simulink model "TestWindRacingSimpleDynamicModelRealForce"  (R2022b)
settings: Solver=FixedStepAuto  StartTime=0.0  StopTime=137  FixedStep=simulator.TimeStep  RelTol=1e-3
undefined symbols (not defined in the file): simulator
settings Model: Creator=At  LastModifiedBy=ateay
settings SolverCC: ConcurrentTasks=on  AlgebraicLoopSolver=TrustRegion  InsertRTBMode=Never (minimum delay)
settings DataIOCC: ReturnWorkspaceOutputs=off
settings DebuggingCC: UnconnectedInputMsg=warning  UnconnectedOutputMsg=warning  UnconnectedLineMsg=warning  SFMachineParentedDataDiag=warning  ArithmeticOperatorsInVariantConditions=warning
settings ModelReferenceCC: EnableRefExpFcnMdlSchedulingChecks=on
settings SFSimCC: SimUseLocalCustomCode=off  CustomCodeUndefinedFunction=UseInterfaceOnly
settings RTWCC: RTWUseLocalCustomCode=off
settings CodeAppCC: StateflowObjectComments=on

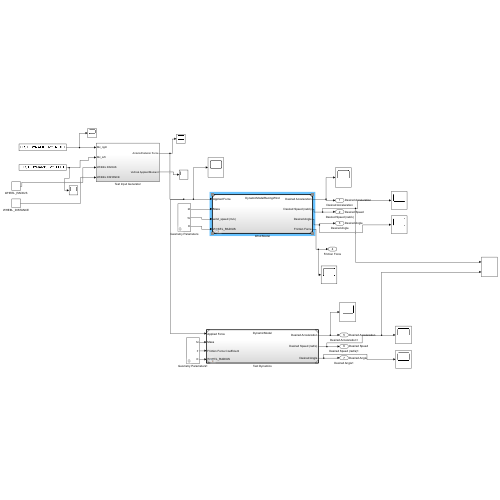
[thumbnail: Simulink's stored preview of the top-level diagram]
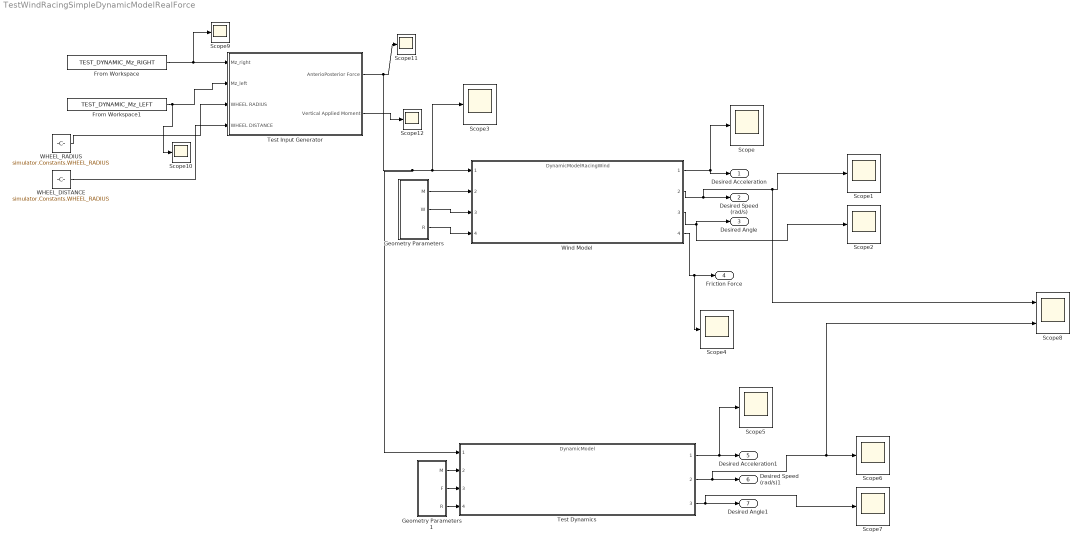
== system TestWindRacingSimpleDynamicModelRealForce ==
  From Workspace : FromWorkspace  VariableName=TEST_DYNAMIC_Mz_RIGHT
  From Workspace1 : FromWorkspace  VariableName=TEST_DYNAMIC_Mz_LEFT
  Geometry Parameters : Subsystem  mask{M=simulator.Sim.Dynamics.Mass, W=simulator.Sim.Dynamics.wind_speed, rR=simulator.Constants.WHEEL_RADIUS}
      mask prompts: M "Mass"; W "Wind"; rR "Radius"
      mask TypeOptions M: Mass/Value
      mask TypeOptions rR: rR/Value
  Geometry Parameters1 : Subsystem  mask{M=98, F=0.0138, rR=0.350}
      mask prompts: M "Mass"; F "Friction"; rR "Radius"
      mask TypeOptions M: Mass/Value
      mask TypeOptions F: Friction/Value
      mask TypeOptions rR: rR/Value
  Scope{,1..7,9..12} (12 alike) : Scope
  Scope8 : Scope  NumInputPorts=2
  "Test Dynamics " : ModelReference  ModelNameDialog=DynamicModel.slx  SimulationMode=Normal  ModelReferenceVersion=1.2
  Test Input Generator : Subsystem
  WHEEL_DISTANCE : Constant  Value=simulator.Constants.WHEEL_RADIUS
  WHEEL_RADIUS : Constant  Value=simulator.Constants.WHEEL_RADIUS
  Wind Model : ModelReference  ModelNameDialog=DynamicModelRacingWind.slx  SimulationMode=Normal  ModelReferenceVersion=1.17
  Desired Acceleration : Outport  SignalName=Desired Acceleration
  Desired Speed (rad/s) : Outport  Port=2  SignalName=Desired Speed
  Desired Angle : Outport  Port=3  SignalName=Desired Angle
  Friction Force : Outport  Port=4
  Desired Acceleration1 : Outport  Port=5  SignalName=Desired Acceleration
  Desired Speed (rad/s)1 : Outport  Port=6  SignalName=Desired Speed
  Desired Angle1 : Outport  Port=7  SignalName=Desired Angle
  wires:
  Wind Model/3 -> Desired Angle/1, Scope2/1
  Wind Model/2 -> Scope8/1, Scope1/1, Desired Speed (rad/s)/1
  Wind Model/1 -> Desired Acceleration/1, Scope/1
  Geometry Parameters/1(M) -> Wind Model/2
  Geometry Parameters/2(W) -> Wind Model/3
  Geometry Parameters/3(R) -> Wind Model/4
  Wind Model/4 -> Scope4/1, Friction Force/1
  Test Input Generator/1(AnterioPosterior Force) -> "Test Dynamics "/1, Wind Model/1, Scope3/1, Scope11/1
  "Test Dynamics "/3 -> Scope7/1, Desired Angle1/1
  "Test Dynamics "/2 -> Scope8/2, Scope6/1, Desired Speed (rad/s)1/1
  "Test Dynamics "/1 -> Scope5/1, Desired Acceleration1/1
  Geometry Parameters1/1(M) -> "Test Dynamics "/2
  Geometry Parameters1/2(F) -> "Test Dynamics "/3
  Geometry Parameters1/3(R) -> "Test Dynamics "/4
  WHEEL_RADIUS/1 -> Test Input Generator/3(WHEEL RADIUS)
  WHEEL_DISTANCE/1 -> Test Input Generator/4(WHEEL DISTANCE)
  Test Input Generator/2(Vertical Applied Moment) -> Scope12/1
  From Workspace/1 -> Scope9/1, Test Input Generator/1(Mz_right)
  From Workspace1/1 -> Scope10/1, Test Input Generator/2(Mz_left)

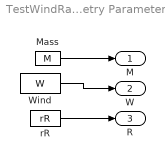
== system TestWindRacingSimpleDynamicModelRealForce/Geometry Parameters ==
  Mass : Constant  Value=M
  Wind : Constant  Value=W
  rR : Constant  Value=rR
  M : Outport
  W : Outport  Port=2
  R : Outport  Port=3
  wires:
  Wind/1 -> W/1
  Mass/1 -> M/1
  rR/1 -> R/1

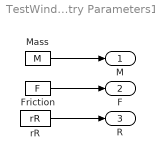
== system TestWindRacingSimpleDynamicModelRealForce/Geometry Parameters1 ==
  Friction : Constant  Value=F
  Mass : Constant  Value=M
  rR : Constant  Value=rR
  M : Outport
  F : Outport  Port=2
  R : Outport  Port=3
  wires:
  Friction/1 -> F/1
  Mass/1 -> M/1
  rR/1 -> R/1

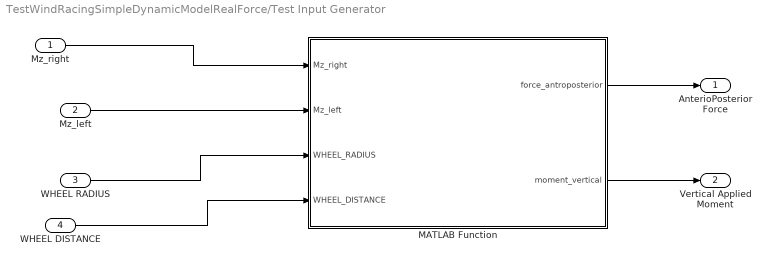
== system TestWindRacingSimpleDynamicModelRealForce/Test Input Generator ==
  Mz_right : Inport
  Mz_left : Inport  Port=2
  WHEEL RADIUS : Inport  Port=3
  WHEEL DISTANCE : Inport  Port=4
  MATLAB Function : MATLAB Function  TreatAsAtomicUnit=on
  AnterioPosterior Force : Outport
  Vertical Applied Moment : Outport  Port=2
  wires:
  Mz_right/1 -> MATLAB Function/1(Mz_right)
  Mz_left/1 -> MATLAB Function/2(Mz_left)
  WHEEL RADIUS/1 -> MATLAB Function/3(WHEEL_RADIUS)
  WHEEL DISTANCE/1 -> MATLAB Function/4(WHEEL_DISTANCE)
  MATLAB Function/1(force_antroposterior) -> AnterioPosterior Force/1
  MATLAB Function/2(moment_vertical) -> Vertical Applied Moment/1

== matlab function TestWindRacingSimpleDynamicModelRealForce/Test Input Generator/MATLAB Function ==
  data: Mz_right input; Mz_left input; WHEEL_RADIUS input; force_antroposterior output; WHEEL_DISTANCE input; moment_vertical output
function [force_antroposterior,moment_vertical]=Force_Conversion(Mz_right, Mz_left,WHEEL_RADIUS,WHEEL_DISTANCE)

%% This function estimates the force and moment applied at the position of installed force cell,...
...based on the moment applied on the right and left instrumented wheels
    
force_antroposterior=(Mz_right/WHEEL_RADIUS)+(Mz_left/WHEEL_RADIUS);
moment_vertical=((Mz_left/WHEEL_RADIUS)-(Mz_right/WHEEL_RADIUS))*(WHEEL_DISTANCE/2);
